simulink model "PropulsionSegmentation"  (R2022a)
settings: Solver=FixedStepAuto  StartTime=0.0  StopTime=30  FixedStep=1e-3  RelTol=1e-3
undefined symbols (not defined in the file or in its folder): phi, r, sigbuilder_block, theta
libraries: robotgazebolib x9, robotlib x8, simulink x4, slpidlib x1
settings Model: Creator=abiyyumufti  LastModifiedBy=abiyyumufti

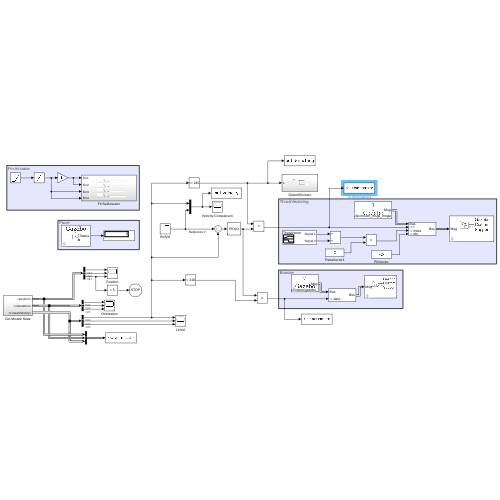
[thumbnail: Simulink's stored preview of the top-level diagram]
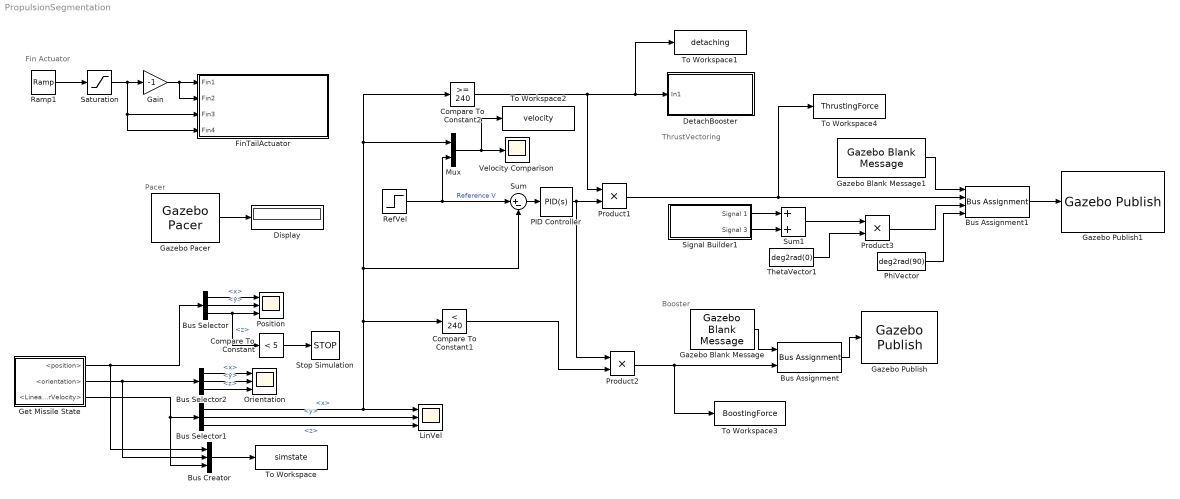
== system PropulsionSegmentation ==
  note: ThrustVectoring
  note: Booster
  note: Fin Actuator
  note: Pacer
  Bus Assignment : BusAssignment  AssignedSignals=data
  Bus Assignment1 : BusAssignment  AssignedSignals=r,theta,phi
  Bus Creator : BusCreator  Inputs=3
  Bus Selector : BusSelector  OutputSignals=x,y,z
  Bus Selector1 : BusSelector  OutputSignals=x,y,z
  Bus Selector2 : BusSelector  OutputSignals=x,y,z
  Compare To Constant : simulink/Logic and Bit Operations/Compare To Constant  relop=<  const=5  OutDataTypeStr=boolean
  Compare To Constant1 : simulink/Logic and Bit Operations/Compare To Constant  relop=<  const=240  OutDataTypeStr=boolean
  Compare To Constant2 : simulink/Logic and Bit Operations/Compare To Constant  relop=>=  const=240  OutDataTypeStr=boolean
  DetachBooster : Subsystem
  Display : Display
  FinTailActuator : Subsystem
  Gain : Gain  Gain=-1
  Gazebo Blank Message : robotgazebolib/Gazebo Blank Message  msgType=gazebo_msgs/custom/gazebo_msgs/Double  sampleTime=0.001  busName='Gazebo_SL_Bus_gazebo_msgs_custom_gazebo_msgs_Double'
      settings: SourceProductBaseCode=RO
  Gazebo Blank Message1 : robotgazebolib/Gazebo Blank Message  msgType=gazebo_msgs/custom/ssm_msgs_msgs/SphericalVector  sampleTime=0.001  busName='Gazebo_SL_Bus_gazebo_msgs_custom_ssm_msgs_msgs_SphericalVector'
      settings: SourceProductBaseCode=RO
  Gazebo Pacer : robotgazebolib/Gazebo Pacer  ResetBehavior=Reset Gazebo simulation time and scene  SampleTime=0.001
      settings: SourceProductBaseCode=RO
  Gazebo Publish : robotgazebolib/Gazebo Publish  topicSource=Specify your own  topic=/gazebo/my_world/booster_force  messageType=gazebo_msgs/custom/gazebo_msgs/Double  sampleTime=0.001
      settings: SourceProductBaseCode=RO
  Gazebo Publish1 : robotgazebolib/Gazebo Publish  topicSource=Specify your own  topic=/gazebo/my_world/thrust_force  messageType=gazebo_msgs/custom/ssm_msgs_msgs/SphericalVector  sampleTime=0.001
      settings: SourceProductBaseCode=RO
  Get Missile State : Subsystem
  LinVel : Scope  NumInputPorts=3
  Mux : Mux  Inputs=2
  Orientation : Scope  NumInputPorts=3
  PID Controller : slpidlib/PID Controller  Controller=PID  Form=Parallel  TimeDomain=Continuous-time  UseExternalTs=off  SampleTime=-1  IntegratorMethod=Forward Euler  FilterMethod=Forward Euler  ControllerParametersSource=internal  P=1000  I=0  UseKiTs=off  D=15  N=100  UseFilter=on  TunerSelectOption=Transfer Function Based (PID Tuner App)  InitialConditionSource=internal  InitialConditionForIntegrator=0  InitialConditionForFilter=0  DifferentiatorICPrevScaledInput=0  ExternalReset=none  TrackingMode=off  Kt=1  LimitOutput=off  SatLimitsSource=internal  UpperSaturationLimit=inf  LowerSaturationLimit=-inf  LinearizeAsGain=on  AntiWindupMode=none  Kb=1  POutMin=[]  POutMax=[]  IOutMin=[]  IOutMax=[]  DOutMin=[]  DOutMax=[]  NOutMin=[]  NOutMax=[]  SumOutMin=[]  SumOutMax=[]  SaturationOutMin=[]  SaturationOutMax=[]  PParamMin=[]  PParamMax=[]  IParamMin=[]  IParamMax=[]  DParamMin=[]  DParamMax=[]  NParamMin=[]  NParamMax=[]  KbParamMin=[]  KbParamMax=[]  KtParamMin=[]  KtParamMax=[]  KbOutMin=[]  KbOutMax=[]  KtOutMin=[]  KtOutMax=[]  IntegratorOutMin=[]  IntegratorOutMax=[]  FilterOutMin=[]  FilterOutMax=[]  SumI1OutMin=[]  SumI1OutMax=[]  SumI2OutMin=[]  SumI2OutMax=[]  SumI3OutMin=[]  SumI3OutMax=[]  SumI4OutMin=[]  SumI4OutMax=[]  SumDOutMin=[]  SumDOutMax=[]  DifferentiatorOutMin=[]  DifferentiatorOutMax=[]  FilterDiffOutCoefMin=[]  FilterDiffOutCoefMax=[]  ReciprocalOutMin=[]  ReciprocalOutMax=[]  SumDenOutMin=[]  SumDenOutMax=[]  SumNumOutMin=[]  SumNumOutMax=[]  DivideOutMin=[]  DivideOutMax=[]  UdiffTsProdOutMin=[]  UdiffTsProdOutMax=[]  NTsProdOutMin=[]  NTsProdOutMax=[]  UintegralTsProdOutMin=[]  UintegralTsProdOutMax=[]  UngainTsProdOutMin=[]  UngainTsProdOutMax=[]  IntegratorContinuousStateAttributes=''  IntegratorStateMustResolveToSignalObject=off  IntegratorRTWStateStorageClass=Auto  FilterContinuousStateAttributes=''  FilterStateMustResolveToSignalObject=off  FilterRTWStateStorageClass=Auto  ParallelPVariant=InternalParameters  IdealPVariant=Disabled  IVariant=InternalParameters  DVariant=InternalParameters  IntegratorVariant=Continuous  SatVariant=Disabled  AWVariant=Passthrough  PCopyVariant=Disabled  TRVariant=Disabled  FdbkBlocksVariant=Forward  IdealPFdbkVariant=Disabled  SatFdbkVariant=Disabled  DerivativeFilterVariant=ContFilter  NVariant=InternalParameters  NCopyVariant=Disabled  FilterICVariant=InternalICsFilter  IntegratorICVariant=InternalICs  ExternalResetVariant=Disabled  TRSumVariant=Passthrough  SumFdbkVariant=Disabled  SumVariant=Sum_PID  TsampFilterVariant=InternalTs  TsampNgainVariant=Passthrough  TsampIntegralVariant=Passthrough  ExternalSaturationOutDataTypeStr=Inherit: Same as second input  aMode=0
  PhiVector : Constant  Value=deg2rad(90)
  Position : Scope  NumInputPorts=3
  Product1 : Product
  Product2 : Product
  Product3 : Product
  Ramp1 : simulink/Sources/Ramp  slope=-deg2rad(20)/5  start=10  InitialOutput=0
  RefVel : Step  Time=1e-3  After=250  SampleTime=0
  Saturation : Saturate  UpperLimit=deg2rad(10)  LowerLimit=-deg2rad(10)
  Signal Builder1 : Subsystem  Tag=STV Subsys  LoadFcn=sigbuilder_block('load');  StartFcn=sigbuilder_block('start');  StopFcn=sigbuilder_block('stop');  ClipboardFcn=sigbuilder_block('clipboard');  mask(Sigbuilder block){tuvar=[0:10]}
      mask help: Simulink:masks:SigbuilderBlock_MD
      mask init:
      | if ~strcmp(get_param(bdroot(gcbh),'SimulationStatus'),'stopped') tuvar = sigbuilder_block('maskInit'); end
      settings: CopyFcn=sigbuilder_block('copy');  DeleteFcn=sigbuilder_block('delete');  ModelCloseFcn=sigbuilder_block('modelClose');  PreSaveFcn=sigbuilder_block('preSave');  PauseFcn=sigbuilder_block('pause');  ContinueFcn=sigbuilder_block('continue');  NameChangeFcn=sigbuilder_block('namechange');  OpenFcn=sigbuilder_block('open',[40.5 0 1399.5 612 ]);  CloseFcn=sigbuilder_block('close');
      mask Display: plot(0, 0, 100, 100,[2, 2, 32, 32, 2], [68, 8, 8, 68, 68],[32, 2], [38, 38], [32, 19, 2],[53, 60, 44], [32, 17, 17, 2],[16, 16, 31, 31]);txt = getActiveGroup(gcbh);text(2, 100, txt,'verticalAlignment', 'top');
  Stop Simulation : Stop
  Sum : Sum  Inputs=|+-
  Sum1 : Sum
  ThetaVector1 : Constant  Value=deg2rad(0)
  To Workspace : ToWorkspace  VariableName=simstate  SaveFormat=Timeseries  SampleTime=-1
  To Workspace1 : ToWorkspace  VariableName=detaching  SaveFormat=Timeseries  SampleTime=-1
  To Workspace2 : ToWorkspace  VariableName=velocity  SaveFormat=Timeseries  SampleTime=-1
  To Workspace3 : ToWorkspace  VariableName=BoostingForce  SaveFormat=Timeseries  SampleTime=-1
  To Workspace4 : ToWorkspace  VariableName=ThrustingForce  SaveFormat=Timeseries  SampleTime=-1
  Velocity Comparison : Scope
  wires:
  Gazebo Pacer/1 -> Display/1
  RefVel/1 -> Mux/2, Sum/1  "Reference V"
  Bus Selector/1 -> Position/1  "<x>"
  Bus Selector/2 -> Position/2  "<y>"
  Bus Selector1/1 -> Compare To Constant2/1, Mux/1, Sum/2, Compare To Constant1/1, LinVel/1  "<x>"
  Bus Selector/3 -> Compare To Constant/1, Position/3  "<z>"
  Gain/1 -> FinTailActuator/2(Fin2), FinTailActuator/1(Fin1)
  Saturation/1 -> FinTailActuator/4(Fin4), FinTailActuator/3(Fin3), Gain/1
  Get Missile State/3(<LinearVelocity>) -> Bus Creator/3, Bus Selector1/1
  Bus Selector1/2 -> LinVel/2  "<y>"
  Bus Selector2/3 -> Orientation/3  "<z>"
  Bus Selector2/2 -> Orientation/2  "<y>"
  Bus Selector1/3 -> LinVel/3  "<z>"
  Bus Selector2/1 -> Orientation/1  "<x>"
  Get Missile State/2(<orientation>) -> Bus Selector2/1, Bus Creator/2
  Ramp1/1 -> Saturation/1
  Mux/1 -> To Workspace2/1, Velocity Comparison/1
  Get Missile State/1(<position>) -> Bus Selector/1, Bus Creator/1
  Sum/1 -> PID Controller/1
  Compare To Constant/1 -> Stop Simulation/1
  Compare To Constant2/1 -> To Workspace1/1, DetachBooster/1(In1), Product1/1
  Bus Assignment/1 -> Gazebo Publish/1
  Gazebo Blank Message/1 -> Bus Assignment/1
  PID Controller/1 -> Product2/1, Product1/2
  Product2/1 -> To Workspace3/1, Bus Assignment/2
  Product1/1 -> To Workspace4/1, Bus Assignment1/2
  PhiVector/1 -> Bus Assignment1/4
  Signal Builder1/2(Signal 3) -> Sum1/2
  Gazebo Blank Message1/1 -> Bus Assignment1/1
  Bus Assignment1/1 -> Gazebo Publish1/1
  ThetaVector1/1 -> Product3/2
  Sum1/1 -> Product3/1
  Signal Builder1/1(Signal 1) -> Sum1/1
  Product3/1 -> Bus Assignment1/3
  Compare To Constant1/1 -> Product2/2
  Bus Creator/1 -> To Workspace/1

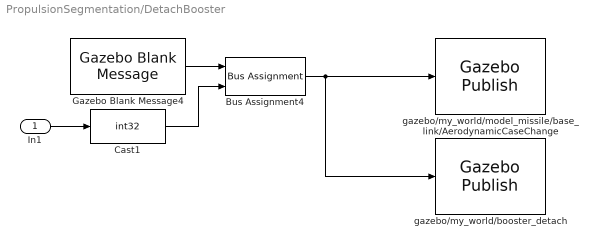
== system PropulsionSegmentation/DetachBooster ==
  In1 : Inport
  Bus Assignment4 : BusAssignment  AssignedSignals=data
  Cast1 : DataTypeConversion  OutDataTypeStr=int32  SaturateOnIntegerOverflow=off  RndMeth=Floor
  Gazebo Blank Message4 : robotgazebolib/Gazebo Blank Message  msgType=gazebo_msgs/custom/gazebo_msgs/Int  sampleTime=0.001  busName='Gazebo_SL_Bus_gazebo_msgs_custom_gazebo_msgs_Int'
      settings: SourceProductBaseCode=RO
  gazebo/my_world/booster_detach : robotgazebolib/Gazebo Publish  topicSource=Specify your own  topic=/gazebo/my_world/booster_detach  messageType=gazebo_msgs/custom/gazebo_msgs/Int  sampleTime=0.001
      settings: SourceProductBaseCode=RO
  gazebo/my_world/model_missile/base_link/AerodynamicCaseChange : robotgazebolib/Gazebo Publish  topicSource=Specify your own  topic=/gazebo/my_world/model_missile/base_link/AerodynamicCaseChange  messageType=gazebo_msgs/custom/gazebo_msgs/Int  sampleTime=0.001
      settings: SourceProductBaseCode=RO
  wires:
  Bus Assignment4/1 -> gazebo/my_world/booster_detach/1, gazebo/my_world/model_missile/base_link/AerodynamicCaseChange/1
  Cast1/1 -> Bus Assignment4/2
  Gazebo Blank Message4/1 -> Bus Assignment4/1
  In1/1 -> Cast1/1

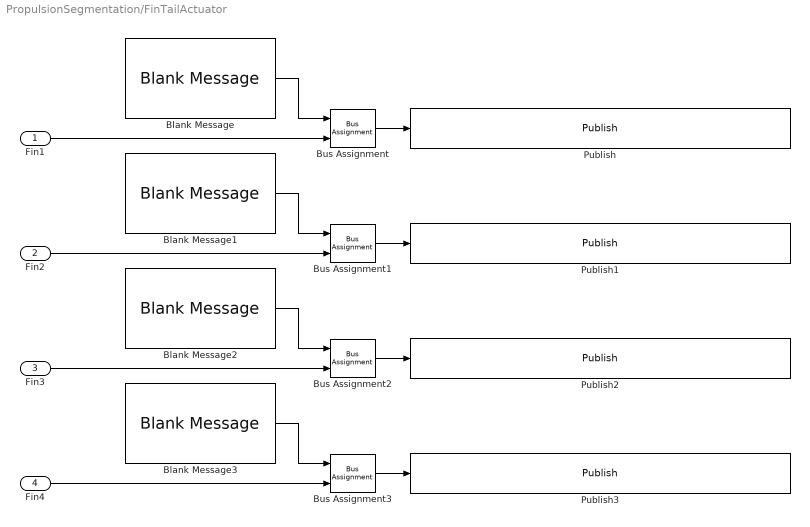
== system PropulsionSegmentation/FinTailActuator ==
  Fin1 : Inport
  Fin2 : Inport  Port=2
  Fin3 : Inport  Port=3
  Fin4 : Inport  Port=4
  Blank Message{,1..3} (4 alike) : robotlib/Blank Message  messageClass=Message  entityType=std_msgs/Float64  messageType=std_msgs/Float64  SampleTime=inf  legacyBusStruct=off
  Bus Assignment{,1..3} (4 alike) : BusAssignment  AssignedSignals=Data
  Publish : robotlib/Publish  topicSource=Select from ROS network  topic=/model_missile_controller/fins_rev1_position_controller/command  messageType=std_msgs/Float64  legacyBusStruct=off  messageQueueLength=1
  Publish1 : robotlib/Publish  topicSource=Select from ROS network  topic=/model_missile_controller/fins_rev2_position_controller/command  messageType=std_msgs/Float64  legacyBusStruct=off  messageQueueLength=1
  Publish2 : robotlib/Publish  topicSource=Select from ROS network  topic=/model_missile_controller/fins_rev3_position_controller/command  messageType=std_msgs/Float64  legacyBusStruct=off  messageQueueLength=1
  Publish3 : robotlib/Publish  topicSource=Select from ROS network  topic=/model_missile_controller/fins_rev4_position_controller/command  messageType=std_msgs/Float64  legacyBusStruct=off  messageQueueLength=1
  wires:
  Fin1/1 -> Bus Assignment/2
  Bus Assignment3/1 -> Publish3/1
  Blank Message/1 -> Bus Assignment/1
  Fin4/1 -> Bus Assignment3/2
  Bus Assignment1/1 -> Publish1/1
  Blank Message3/1 -> Bus Assignment3/1
  Blank Message2/1 -> Bus Assignment2/1
  Bus Assignment/1 -> Publish/1
  Blank Message1/1 -> Bus Assignment1/1
  Bus Assignment2/1 -> Publish2/1
  Fin2/1 -> Bus Assignment1/2
  Fin3/1 -> Bus Assignment2/2

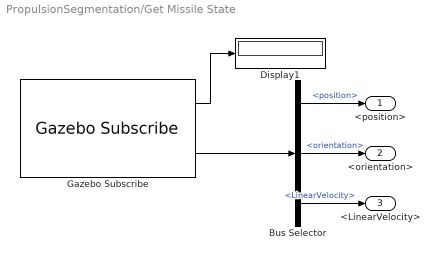
== system PropulsionSegmentation/Get Missile State ==
  Bus Selector : BusSelector  OutputSignals=Pose.position,Pose.orientation,LinearVelocity
  Display1 : Display
  Gazebo Subscribe : robotgazebolib/Gazebo Subscribe  topicSource=From Gazebo  topic=/gazebo/my_world/DynamicState  messageType=gazebo_msgs/custom/ssm_msgs_msgs/DynamicState  sampleTime=0.001
      settings: SourceProductBaseCode=RO
  <position> : Outport
  <orientation> : Outport  Port=2
  <LinearVelocity> : Outport  Port=3
  wires:
  Gazebo Subscribe/2 -> Bus Selector/1
  Gazebo Subscribe/1 -> Display1/1
  Bus Selector/1 -> <position>/1  "<position>"
  Bus Selector/3 -> <LinearVelocity>/1  "<LinearVelocity>"
  Bus Selector/2 -> <orientation>/1  "<orientation>"

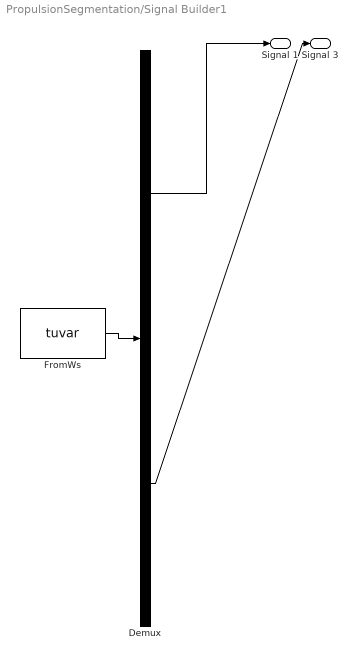
== system PropulsionSegmentation/Signal Builder1 ==
  Demux : Demux  Tag=STV Demux  Outputs=2
      settings: DisplayOption=none
  FromWs : FromWorkspace  Tag=STV FromWs  VariableName=tuvar
      SigBuilderData=|
      | common.afterFinalStr = 'Extrapolate'
      | common.sampleTime = 0
      | dataSet.timeRange = [0 60]
      | dataSet.name = 'ThetaVector'
      | sbobj.Groups.Name = 'ThetaVector'
      | sbobj.Groups.Signals(1).Name = 'Signal 1'
      | sbobj.Groups.Signals(1).XData = [0 6 9 12 60]
      | sbobj.Groups.Signals(1).YData = [0 0 1 0 0]
      | sbobj.Groups.Signals(2).Name = 'Signal 3'
      | sbobj.Groups.Signals(2).XData = [0 12 15 18 60]
      | sbobj.Groups.Signals(2).YData = [0 0 -2 0 0]
      | sbobj.Groups.TimeRange = [0 60]
  Signal 1 : Outport  Tag=STV Outport
  Signal 3 : Outport  Tag=STV Outport  Port=2
  wires:
  FromWs/1 -> Demux/1
  Demux/1 -> Signal 1/1
  Demux/2 -> Signal 3/1
